simulink model "Oscillator"  (R2020b)
settings: Solver=FixedStepDiscrete  StartTime=0.0  StopTime=1500.0  FixedStep=1  RelTol=1e-3
settings Model: Creator=ncleju  LastModifiedBy=ncleju

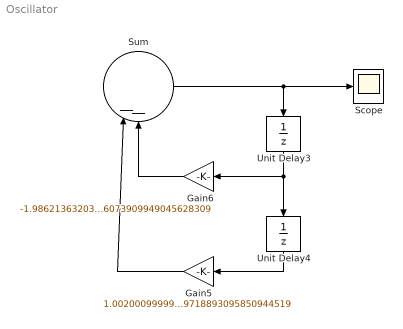
== system Oscillator ==
  Gain5 : Gain  Gain=1.002000999999999919509718893095850944519
  Gain6 : Gain  Gain=-1.986213632031584408466073909949045628309
  Scope : Scope
  Sum : Sum  Inputs=||||||--
  Unit Delay3 : UnitDelay  InitialCondition=1  SampleTime=-1  HasFrameUpgradeWarning=on
  Unit Delay4 : UnitDelay  SampleTime=-1  HasFrameUpgradeWarning=on
  wires:
  Sum/1 -> Scope/1, Unit Delay3/1
  Unit Delay3/1 -> Unit Delay4/1, Gain6/1
  Unit Delay4/1 -> Gain5/1
  Gain6/1 -> Sum/2
  Gain5/1 -> Sum/1
